simulink model "modelext"  (R2017a)
settings: Solver=VariableStepAuto  StartTime=0.0  StopTime=100  RelTol=1e-3
values from neighbouring files (symbols this model uses):
  D1 = Delta(:,:,i)    [HFTC.m]
  DH1 = blkdiag(eye(2),Delta(3:end,3:end,i))    [HFTC.m]
  L = L_FFTC    [HFTC.m]
undefined symbols (not defined in the file or in its folder): A, B, C, Cz
settings Model: Creator=vk1014  LastModifiedBy=vk1014

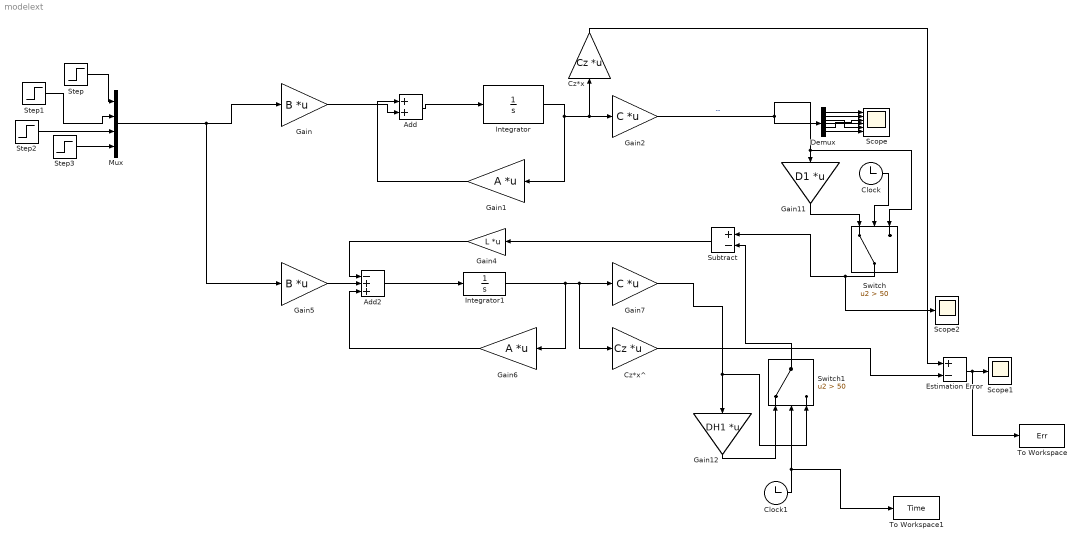
== system modelext ==
  Add : Sum
  Add2 : Sum  Inputs=-++
  Clock : Clock
  Clock1 : Clock
  Cz*x : Gain  Gain=Cz  Multiplication=Matrix(K*u)
  Cz*x^ : Gain  Gain=Cz  Multiplication=Matrix(K*u)
  Demux : Demux  Outputs=6
  Estimation Error : Sum  Inputs=+-
  Gain : Gain  Gain=B  Multiplication=Matrix(K*u)
  Gain1 : Gain  Gain=A  Multiplication=Matrix(K*u)
  Gain11 : Gain  Gain=D1  Multiplication=Matrix(K*u)
  Gain12 : Gain  Gain=DH1  Multiplication=Matrix(K*u)
  Gain2 : Gain  Gain=C  Multiplication=Matrix(K*u)
  Gain4 : Gain  Gain=L  Multiplication=Matrix(K*u)
  Gain5 : Gain  Gain=B  Multiplication=Matrix(K*u)
  Gain6 : Gain  Gain=A  Multiplication=Matrix(K*u)
  Gain7 : Gain  Gain=C  Multiplication=Matrix(K*u)
  Integrator : Integrator  InitialCondition=1
  Integrator1 : Integrator  InitialCondition=1
  Mux : Mux
  Scope : Scope  NumInputPorts=6
  Scope1 : Scope
  Scope2 : Scope
  Step{,1..3} (4 alike) : Step  SampleTime=0
  Subtract : Sum  Inputs=+-
  Switch : Switch  Criteria=u2 > Threshold  Threshold=50
  Switch1 : Switch  Criteria=u2 > Threshold  Threshold=50
  To Workspace : ToWorkspace  VariableName=Err  SampleTime=-1
      settings: Save2DSignal=2-D array (concatenate along first dimension)
  To Workspace1 : ToWorkspace  VariableName=Time  SampleTime=-1
      settings: Save2DSignal=2-D array (concatenate along first dimension)
  wires:
  Switch1/1 -> Subtract/2
  Gain7/1 -> Switch1/3, Gain12/1
  Gain12/1 -> Switch1/1
  Mux/1 -> Gain5/1, Gain/1
  Clock1/1 -> To Workspace1/1, Switch1/2
  Switch/1 -> Scope2/1, Subtract/1
  Clock/1 -> Switch/2
  Demux/1 -> Scope/1
  Add2/1 -> Integrator1/1
  Gain11/1 -> Switch/1
  Gain/1 -> Add/2
  Demux/3 -> Scope/5
  Step1/1 -> Mux/2
  Cz*x/1 -> Estimation Error/1
  Step3/1 -> Mux/4
  Step2/1 -> Mux/3
  Gain5/1 -> Add2/2
  Estimation Error/1 -> To Workspace/1, Scope1/1
  Gain6/1 -> Add2/3
  Subtract/1 -> Gain4/1
  Gain2/1 -> Switch/3, Gain11/1, Demux/1  "--"
  Integrator1/1 -> Gain6/1, Cz*x^/1, Gain7/1
  Demux/2 -> Scope/2
  Add/1 -> Integrator/1
  Integrator/1 -> Cz*x/1, Gain2/1, Gain1/1
  Step/1 -> Mux/1
  Cz*x^/1 -> Estimation Error/2
  Gain4/1 -> Add2/1
  Demux/4 -> Scope/4
  Demux/5 -> Scope/3
  Demux/6 -> Scope/6
  Gain1/1 -> Add/1
